simulink model "LFC_Fuzzy_AREA1"  (R2021a)
settings: Solver=VariableStepAuto  StartTime=0.0  StopTime=25  RelTol=1e-3
libraries: fuzblock x1, pid_lib x1, spspowerguiLib x1
settings Model: Creator=B.HARISH  LastModifiedBy=B.HARISH

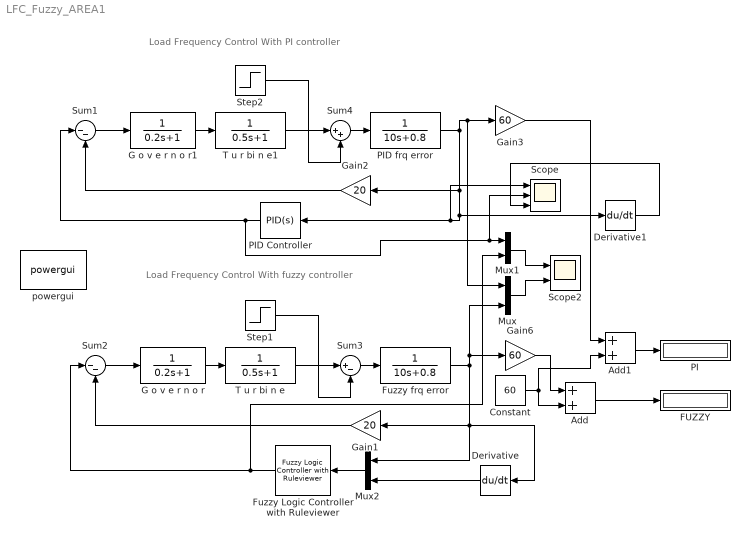
== system LFC_Fuzzy_AREA1 ==
  note: Load Frequency Control With fuzzy controller
  note: Load Frequency Control With PI controller
  Add : Sum
  Add1 : Sum
  Constant : Constant  Value=60
  Derivative : Derivative
  Derivative1 : Derivative
  FUZZY : Display
  Fuzzy Logic Controller with Ruleviewer : fuzblock/Fuzzy Logic  Controller  with Ruleviewer  fismatrix=LFC_A1_1  Ts=2
  Fuzzy frq error : TransferFcn  Denominator=[10 0.8]
  G o v e r n o r : TransferFcn  Denominator=[0.2 1]
  G o v e r n o r1 : TransferFcn  Denominator=[0.2 1]
  Gain1 : Gain  Gain=20
  Gain2 : Gain  Gain=20
  Gain3 : Gain  Gain=60
  Gain6 : Gain  Gain=60
  Mux : Mux  Inputs=2
  Mux1 : Mux  Inputs=2
  Mux2 : Mux  Inputs=2
  PI : Display
  PID Controller : pid_lib/PID Controller  Controller=PID  Form=Parallel  TimeDomain=Continuous-time  UseExternalTs=off  SampleTime=-1  IntegratorMethod=Forward Euler  FilterMethod=Forward Euler  ControllerParametersSource=internal  P=0  I=7  D=0  UseFilter=on  N=100  TunerSelectOption=Transfer Function Based (PID Tuner App)  InitialConditionSource=internal  InitialConditionForIntegrator=0  InitialConditionForFilter=0  DifferentiatorICPrevScaledInput=0  ExternalReset=none  TrackingMode=off  Kt=1  LimitOutput=off  SatLimitsSource=internal  UpperSaturationLimit=inf  LowerSaturationLimit=-inf  LinearizeAsGain=on  AntiWindupMode=none  Kb=1  POutMin=[]  POutMax=[]  IOutMin=[]  IOutMax=[]  DOutMin=[]  DOutMax=[]  NOutMin=[]  NOutMax=[]  SumOutMin=[]  SumOutMax=[]  SaturationOutMin=[]  SaturationOutMax=[]  PParamMin=[]  PParamMax=[]  IParamMin=[]  IParamMax=[]  DParamMin=[]  DParamMax=[]  NParamMin=[]  NParamMax=[]  KbParamMin=[]  KbParamMax=[]  KtParamMin=[]  KtParamMax=[]  KbOutMin=[]  KbOutMax=[]  KtOutMin=[]  KtOutMax=[]  IntegratorOutMin=[]  IntegratorOutMax=[]  FilterOutMin=[]  FilterOutMax=[]  SumI1OutMin=[]  SumI1OutMax=[]  SumI2OutMin=[]  SumI2OutMax=[]  SumI3OutMin=[]  SumI3OutMax=[]  SumI4OutMin=[]  SumI4OutMax=[]  SumDOutMin=[]  SumDOutMax=[]  DifferentiatorOutMin=[]  DifferentiatorOutMax=[]  FilterDiffOutCoefMin=[]  FilterDiffOutCoefMax=[]  ReciprocalOutMin=[]  ReciprocalOutMax=[]  SumDenOutMin=[]  SumDenOutMax=[]  SumNumOutMin=[]  SumNumOutMax=[]  DivideOutMin=[]  DivideOutMax=[]  UdiffTsProdOutMin=[]  UdiffTsProdOutMax=[]  NTsProdOutMin=[]  NTsProdOutMax=[]  UintegralTsProdOutMin=[]  UintegralTsProdOutMax=[]  UngainTsProdOutMin=[]  UngainTsProdOutMax=[]  IntegratorContinuousStateAttributes=''  IntegratorStateMustResolveToSignalObject=off  IntegratorRTWStateStorageClass=Auto  FilterContinuousStateAttributes=''  FilterStateMustResolveToSignalObject=off  FilterRTWStateStorageClass=Auto  ParallelPVariant=InternalParameters  IdealPVariant=Disabled  IVariant=InternalParameters  DVariant=InternalParameters  IntegratorVariant=Continuous  SatVariant=Disabled  AWVariant=Passthrough  PCopyVariant=Disabled  TRVariant=Disabled  FdbkBlocksVariant=Forward  IdealPFdbkVariant=Disabled  SatFdbkVariant=Disabled  DerivativeFilterVariant=ContFilter  NVariant=InternalParameters  NCopyVariant=Disabled  FilterICVariant=InternalICsFilter  IntegratorICVariant=InternalICs  ExternalResetVariant=Disabled  TRSumVariant=Passthrough  SumFdbkVariant=Disabled  SumVariant=Sum_PID  TsampFilterVariant=InternalTs  TsampNgainVariant=Passthrough  TsampIntegralVariant=Passthrough  ExternalSaturationOutDataTypeStr=Inherit: Same as second input
  PID frq error : TransferFcn  Denominator=[10 0.8]
  Scope : Scope  NumInputPorts=3
  Scope2 : Scope  NumInputPorts=2
  Step1 : Step  Time=0  After=0.2  SampleTime=0
  Step2 : Step  Time=0  After=-0.2  SampleTime=0
  Sum1 : Sum  Inputs=|--
  Sum2 : Sum  Inputs=|--
  Sum3 : Sum  Inputs=|+-
  Sum4 : Sum  Inputs=|++
  T u r bi n e : TransferFcn  Denominator=[0.5 1]
  T u r bi n e1 : TransferFcn  Denominator=[0.5 1]
  powergui : spspowerguiLib/powergui  Priority=1  SimulationMode=Continuous  SampleTime=50e-6  frequency=60  Iterations=50  frequencyindice=60  Pbase=100e6  ErrMax=1e-4  UnitsV=kV  UnitsW=MW  buscounter=0  FunctionMessages=off  echomessages=off  EnableUseOfTLC=off  CurrentSourceSwitches=off  DisableSnubberDevices=off  DisableRonSwitches=off  DisableVfSwitches=off  DisplayEquations=off  AutomaticDiscreteSolvers=off  SolverType=Tustin/Backward Euler (TBE)  Interpol=off  ExternalGateDelay=off  methode=off  Ts=100  x0status=blocks  SPID=off  SwTol=0  HookPort=off  NonlinearTolerance=1e-4  nMaxIteration=100  ContinueOnMaxIteration=off  RestoreLinks=warning  ResistiveCurrentMeasurement=off  Frange=[0:2:500]  Ylog=off  Xlog=on  ShowGrid=off  save=off  variable=ZData  structure=0  ZoomFFT=off  StartTime=0.0  cycles=1  DisplayStyle=1  fundamental=60  FreqAxis=off  MaxFrequency=1000  frequencyindicesteady=1  RmsSteady=1  display=off
  wires:
  Fuzzy Logic Controller with Ruleviewer/1 -> Mux1/2, Sum2/1
  Gain1/1 -> Sum2/2
  Fuzzy frq error/1 -> Gain6/1, Mux/2, Gain1/1, Derivative/1, Mux2/1
  Sum3/1 -> Fuzzy frq error/1
  T u r bi n e/1 -> Sum3/1
  Sum2/1 -> G o v e r n o r/1
  Step1/1 -> Sum3/2
  G o v e r n o r/1 -> T u r bi n e/1
  PID Controller/1 -> Scope/2, Mux1/1, Sum1/1
  Gain2/1 -> Sum1/2
  PID frq error/1 -> Mux/1, Gain3/1, Derivative1/1, PID Controller/1, Scope/1, Gain2/1
  Sum4/1 -> PID frq error/1
  T u r bi n e1/1 -> Sum4/1
  Sum1/1 -> G o v e r n o r1/1
  Step2/1 -> Sum4/2
  G o v e r n o r1/1 -> T u r bi n e1/1
  Mux1/1 -> Scope2/1
  Mux/1 -> Scope2/2
  Mux2/1 -> Fuzzy Logic Controller with Ruleviewer/1
  Derivative/1 -> Mux2/2
  Derivative1/1 -> Scope/3
  Add/1 -> FUZZY/1
  Gain6/1 -> Add/1
  Add1/1 -> PI/1
  Gain3/1 -> Add1/1
  Constant/1 -> Add/2, Add1/2
